simulink model "TEST_HIL"  (R2020a)
settings: Solver=FixedStepAuto  StartTime=0.0  StopTime=10  FixedStep=0.001  RelTol=1e-3
undefined symbols (not defined in the file): serial, Ts
libraries: instrumentlib x3, etargetslib x1
settings Model: Creator=Noxi-PC  LastModifiedBy=Noxi-PC

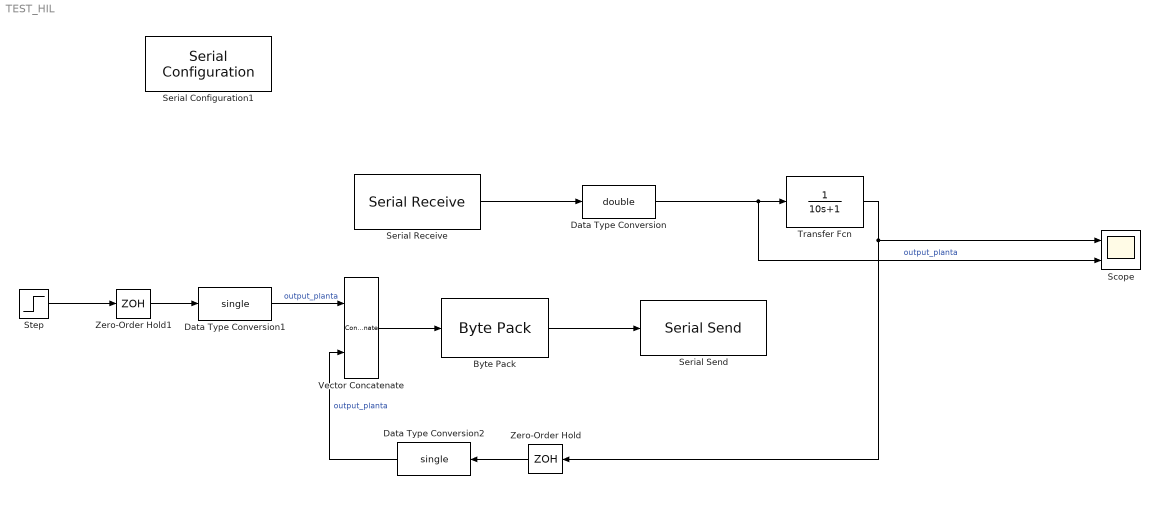
== system TEST_HIL ==
  Byte Pack : etargetslib/Byte Pack  datatypes={'single'}  byteAlign=4
  Data Type Conversion : DataTypeConversion  OutDataTypeStr=double
  Data Type Conversion1 : DataTypeConversion  OutDataTypeStr=single
  Data Type Conversion2 : DataTypeConversion  OutDataTypeStr=single
  Scope : Scope  NumInputPorts=2
  Serial Configuration1 : instrumentlib/Serial Configuration  Priority=-200000  ComPortMenu=COM6  ComPort=COM6  ObjConstructor=serial('COM6');  BaudRate=115200  DataBits=8  Parity=none  StopBits=1  FlowControl=none  Timeout=10  ByteOrder=LittleEndian
  Serial Receive : instrumentlib/Serial Receive  ComPortMenu=COM6  ComPort=COM6  ObjConstructor=serial('COM6');  Terminator=<none>  DataSize="[1  1]"  DataType=single  EnableBlockingMode=on  ActionDataUnavailable=Output last received value  CustomValue=0  SampleTime=Ts
  Serial Send : instrumentlib/Serial Send  ComPortMenu=COM6  ComPort=COM6  ObjConstructor=serial('COM6');  Terminator=<none>  EnableBlockingMode=on
  Step : Step  Time=0  After=2  SampleTime=0
  Transfer Fcn : TransferFcn  Denominator=[10 1]
  Vector Concatenate : Concatenate
  Zero-Order Hold : ZeroOrderHold  SampleTime=Ts
  Zero-Order Hold1 : ZeroOrderHold  SampleTime=Ts
  wires:
  Zero-Order Hold1/1 -> Data Type Conversion1/1
  Data Type Conversion/1 -> Transfer Fcn/1, Scope/2  "output_planta"
  Step/1 -> Zero-Order Hold1/1
  Byte Pack/1 -> Serial Send/1
  Transfer Fcn/1 -> Scope/1, Zero-Order Hold/1
  Vector Concatenate/1 -> Byte Pack/1
  Data Type Conversion1/1 -> Vector Concatenate/1  "output_planta"
  Zero-Order Hold/1 -> Data Type Conversion2/1
  Data Type Conversion2/1 -> Vector Concatenate/2  "output_planta"
  Serial Receive/1 -> Data Type Conversion/1
